simulink model "PartTwo"  (R2025b)
settings: Solver=VariableStepAuto  StartTime=0.0  StopTime=t_end  RelTol=1e-3
values from neighbouring files (symbols this model uses):
  t_sample = 0.0000001    (= 1e-07)    [HomeExamenPArtTwo.m]
libraries: cstblocks x2
settings Model: Creator=Jorben  LastModifiedBy=Jorben

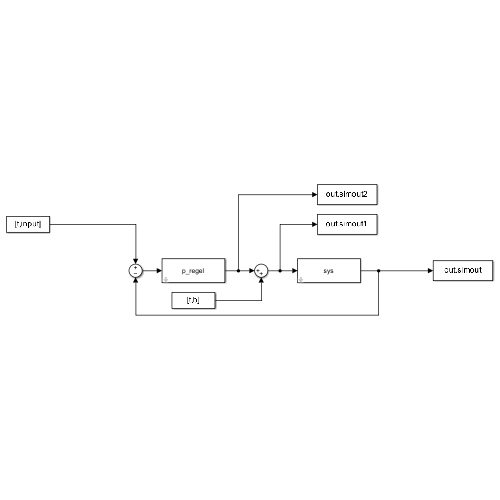
[thumbnail: Simulink's stored preview of the top-level diagram]
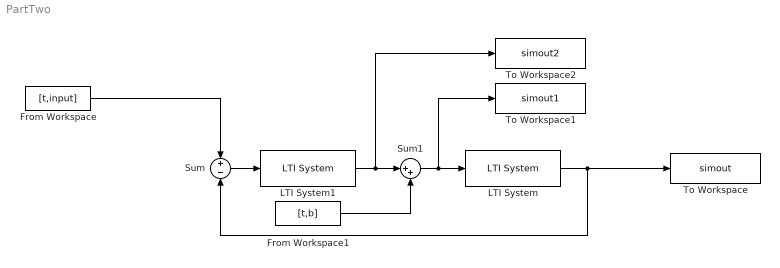
== system PartTwo ==
  From Workspace : FromWorkspace  VariableName=[t,input]  SampleTime=t_sample
  From Workspace1 : FromWorkspace  VariableName=[t,b]  SampleTime=t_sample
  LTI System : cstblocks/LTI System  sys=sys  IC=[]  PadeOrder=0
  LTI System1 : cstblocks/LTI System  sys=p_regel  IC=[]  PadeOrder=0
  Sum : Sum  Inputs=+-
  Sum1 : Sum  Inputs=|++
  To Workspace : ToWorkspace  VariableName=simout  SampleTime=t_sample
  To Workspace1 : ToWorkspace  VariableName=simout1  SampleTime=t_sample
  To Workspace2 : ToWorkspace  VariableName=simout2  SampleTime=t_sample
  wires:
  From Workspace/1 -> Sum/1
  Sum/1 -> LTI System1/1
  LTI System/1 -> Sum/2, To Workspace/1
  LTI System1/1 -> To Workspace2/1, Sum1/1
  Sum1/1 -> To Workspace1/1, LTI System/1
  From Workspace1/1 -> Sum1/2
